simulink model "HEV_Model_Local_Solver"  (R2015a)
settings: Solver=ode23t  StartTime=0.0  StopTime=195  RelTol=1e-5  AbsTol=1e-4
PreLoadFcn:
  | load UrbanCycle1
  | load UrbanCycle2
  | load UrbanCycle3
  | load UrbanCycle4
  | load UrbanCycle5
  | 
  | assignin('base','decimation',1)
  | Pbatt = 21e3;
  | Vbatt =100;
  | Ts = 6e-5;   % time step
  | 
  | Drive_Cycle_Num = 1;
PostLoadFcn:
  | warning off Simulink:SL_UsingDefaultMaxStepSize
  | warning off Simulink:blocks:MatchingGotoNotFound
  | warning off Simulink:blocks:MatchingFromNotFound
  | warning off Simulink:blocks:TDelayBufferTooSmall
  | warning off Simulink:SL_SaveWithParameterizedLinks_Warning
  | warning off Simulink:SL_TDelayBufferTooSmall
  | warning off ne_sli:nesl_compile:SolverNotRecommended
  | warning off Simulink:SL_OutputNotConnected
  | warning off Simulink:SL_SetParamLinkChangeWarn
  | warning off Simulink:Engine:SaveWithDisabledLinks_Warning
  | warning('off','Simulink:SL_UINotUpdatedDuringRapidAccelSim');
  | warning off Simulink:Engine:OutputNotConnected
  | warning off Simulink:Engine:UINotUpdatedDuringRapidAccelSim
  | warning off Simulink:Engine:SaveWithParameterizedLinks_Warning
  | warning off Simulink:Engine:SolverMaskedZC
  | set_param(bdroot,'MaskedZcDiagnostic','none');
  | warning off Simulink:Engine:SolverInconsistentInitialConditionsWarnForDAE
  | set_param(bdroot,'IgnoredZcDiagnostic','none');
  | warning off Simulink:Engine:SolverIgnoredZCBracketing
  | set_param(bdroot,'MaxConsecutiveZCsMsg','none');
  | warning off Simulink:Engine:SolverConsecutiveZCNum
  | warning off Simulink:Engine:SolverMinStepSizeWarnForDAE
  | warning off Simulink:blocks:TDelayFixedBuffer
  | warning off Simulink:Engine:ExtModeCantUploadDataConstantSampleTime
  | warning off Simulink:tools:extModeOpenXPCWarning
  | warning off xPCTarget:sampleTime:sampleTimeInvariance
  | 
  | 
  | %Setup_HEV_Model_Configurations
InitFcn:
  | %Configure_HEV_Simulation
StartFcn:
  | tic;
StopFcn:
  | Elapsed_Sim_Time = toc; disp(['Elapsed time is ' num2str(Elapsed_Sim_Time)]); disp(['Fuel Used: ' num2str(FuelUsedLiters) ' Liters']); disp(' ');
model workspace (MAT data in the model file):
  guiH = 18054.0001221
undefined symbols (not defined in the file or in its folder): drive_block, drive_enginemodel, HEV_Param, sigbuilder_block, speed, torque
libraries: fl_lib x73, nesl_utility x31, sdl_lib x2, elec_lib x2, simulink x1, HEV_Battery_Lib x1, HEV_Vehicle_Dynamics_Lib x1, powerlib x1, slrtlib x1
(part 2 of 2)

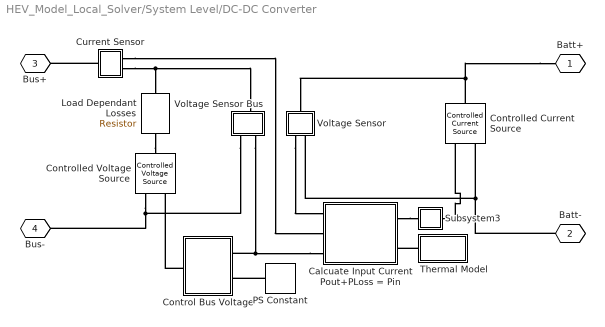
== system HEV_Model_Local_Solver/System Level/DC-DC Converter ==
  Calcuate Input Current Pout+PLoss = Pin : Subsystem
  Control Bus Voltage : Subsystem
  Controlled Current Source : fl_lib/Electrical/Electrical Sources/Controlled Current Source
  Controlled Voltage Source : fl_lib/Electrical/Electrical Sources/Controlled Voltage Source
  Current Sensor : Subsystem
  Load Dependant Losses : fl_lib/Electrical/Electrical Elements/Resistor  R=RLoadLoss Ohm  i_specify=off  i_priority=High  i=0 A  v_specify=off  v_priority=High  v=0 V
  PS Constant : fl_lib/Physical Signals/Sources/PS Constant  constant=Vout
  Subsystem3 : Subsystem
      mask Display: disp('S')
  Thermal Model : Subsystem
  Voltage Sensor : Subsystem
  Voltage Sensor Bus : Subsystem
  " Batt+" : PMIOPort  Tag=PMCPort  Port=1  Side=Left
  " Batt-" : PMIOPort  Tag=PMCPort  Port=2  Side=Left
  " Bus+" : PMIOPort  Tag=PMCPort  Port=3  Side=Right
  " Bus-" : PMIOPort  Tag=PMCPort  Port=4  Side=Right
  connections:
  Thermal Model/LConn1 -- Calcuate Input Current Pout+PLoss = Pin/RConn2
  Calcuate Input Current Pout+PLoss = Pin/LConn3 -- Control Bus Voltage/LConn1 -- Voltage Sensor Bus/RConn2
  Subsystem3/LConn1 -- Controlled Current Source/RConn1
  PS Constant/RConn1 -- Control Bus Voltage/LConn2
  Control Bus Voltage/RConn1 -- Controlled Voltage Source/RConn1
  " Batt+"/RConn1 -- Controlled Current Source/LConn1 -- Voltage Sensor/LConn1
  " Batt-"/RConn1 -- Controlled Current Source/RConn2 -- Voltage Sensor/RConn2
  Load Dependant Losses/RConn1 -- Controlled Voltage Source/LConn1
  " Bus-"/RConn1 -- Controlled Voltage Source/RConn2 -- Voltage Sensor Bus/RConn1
  Current Sensor/LConn1 -- " Bus+"/RConn1
  Current Sensor/RConn2 -- Load Dependant Losses/LConn1 -- Voltage Sensor Bus/LConn1
  Voltage Sensor/RConn1 -- Calcuate Input Current Pout+PLoss = Pin/LConn1
  Current Sensor/RConn1 -- Calcuate Input Current Pout+PLoss = Pin/LConn2
  Calcuate Input Current Pout+PLoss = Pin/RConn1 -- Subsystem3/RConn1

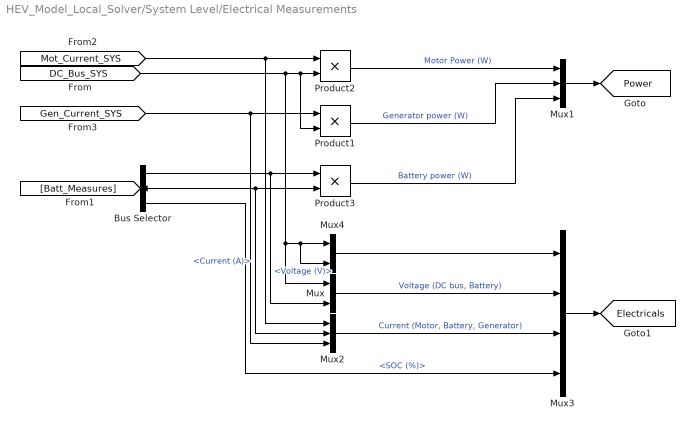
== system HEV_Model_Local_Solver/System Level/Electrical Measurements ==
  Bus Selector : BusSelector  OutputSignals=Voltage (V),Current (A),SOC (%)
  Mux : Mux  Inputs=2
  Mux1 : Mux  Inputs=3
  Mux2 : Mux  Inputs=3
  Mux3 : Mux
  Mux4 : Mux  Inputs=2
  Product1 : Product  RndMeth=Zero
  Product2 : Product  RndMeth=Zero
  Product3 : Product  RndMeth=Zero
  tag scope: Electricals=global, Power=global
  wires:
  Product2/1 -> Mux1/1  "Motor Power (W)"
  Product1/1 -> Mux1/2  "Generator power (W)"
  Product3/1 -> Mux1/3  "Battery power (W)"
  [Mot_Current_SYS] -> Product2/1, Mux2/1
  Mux1/1 -> [Power]
  [Batt_Measures] -> Bus Selector/1
  Bus Selector/1 -> Mux/2, Product3/1  "<Voltage (V)>"
  Bus Selector/2 -> Product3/2, Mux2/2  "<Current (A)>"
  Mux/1 -> Mux3/2  "Voltage (DC bus, Battery)"
  Mux2/1 -> Mux3/3  "Current (Motor, Battery, Generator)"
  [Gen_Current_SYS] -> Product1/1, Mux2/3
  Bus Selector/3 -> Mux3/4  "<SOC (%)>"
  [DC_Bus_SYS] -> Product2/2, Product1/2, Mux/1, Mux4/1, Mux4/2
  Mux3/1 -> [Electricals]
  Mux4/1 -> Mux3/1

== system HEV_Model_Local_Solver/System Level/Generator, Drive Measurements ==
  Constant1 : Constant  Value=0
  Constant2 : Constant  Value=0
  Mux1 : Mux
  Mux2 : Mux
  tag scope: GeneratorDrive=global, MotorDrive=global
  wires:
  [Mot_RPM_SYS] -> Mux2/2
  [Mot_TReq_SYS] -> Mux2/4, Mux2/3
  Mux2/1 -> [MotorDrive]
  Constant2/1 -> Mux2/1
  [Gen_RPM_SYS] -> Mux1/2
  [Gen_TReq_SYS] -> Mux1/3, Mux1/4
  Mux1/1 -> [GeneratorDrive]
  Constant1/1 -> Mux1/1

== system HEV_Model_Local_Solver/System Level/Speed Sensor1 ==
  Ideal Rotational Motion Sensor : fl_lib/Mechanical/Mechanical Sensors/Ideal Rotational Motion Sensor  offset=0 rad
  Mechanical Rotational Reference : fl_lib/Mechanical/Rotational Elements/Mechanical Rotational Reference
  PS-Simulink Converter : nesl_utility/PS-Simulink Converter  PhysicalDomain=network_engine_domain  SubClassName=ps_output  LeftPortType=input  RightPortType=output  PseudoPeriodic=off  Frequencies=[]  Unit=rpm  AffineConversion=off
  Sh : PMIOPort  Port=1  Side=Left
  Sh1 : PMIOPort  Port=2  Side=Right
  tag scope: Mot_RPM_SYS=global
  wires:
  PS-Simulink Converter/1 -> [Mot_RPM_SYS]  "Mot_RPM"
  connections:
  PS-Simulink Converter/LConn1 -- Ideal Rotational Motion Sensor/RConn2
  Sh/RConn1 -- Ideal Rotational Motion Sensor/LConn1 -- Sh1/RConn1
  Ideal Rotational Motion Sensor/RConn1 -- Mechanical Rotational Reference/LConn1

== system HEV_Model_Local_Solver/System Level/Speed Sensor2 ==
  Ideal Rotational Motion Sensor : fl_lib/Mechanical/Mechanical Sensors/Ideal Rotational Motion Sensor  offset=0 rad
  Mechanical Rotational Reference : fl_lib/Mechanical/Rotational Elements/Mechanical Rotational Reference
  PS-Simulink Converter : nesl_utility/PS-Simulink Converter  PhysicalDomain=network_engine_domain  SubClassName=ps_output  LeftPortType=input  RightPortType=output  PseudoPeriodic=off  Frequencies=[]  Unit=rpm  AffineConversion=off
  Sh : PMIOPort  Port=1  Side=Left
  Sh1 : PMIOPort  Port=2  Side=Right
  tag scope: Gen_RPM_SYS=global
  wires:
  PS-Simulink Converter/1 -> [Gen_RPM_SYS]  "Gen_RPM"
  connections:
  Ideal Rotational Motion Sensor/LConn1 -- Sh/RConn1 -- Sh1/RConn1
  PS-Simulink Converter/LConn1 -- Ideal Rotational Motion Sensor/RConn2
  Ideal Rotational Motion Sensor/RConn1 -- Mechanical Rotational Reference/LConn1

== system HEV_Model_Local_Solver/System Level/Synchronous Generator & Drive ==
  note: Note that the generator can turn backwards - this happens when accelerating from rest. The
      | generator also acts as a starter for the engine. If the engine is running, then the generator
      | controller is used to manage battery charging using torque-control mode, otherwise the
      | generator controller controls generator speed.
  TReq : Inport
  Calculate mechanical power & torque : Subsystem
      mask Display: disp('S')
  Calculate power : Subsystem
      mask Display: disp('S')
  GF : Subsystem
      mask Display: disp('GF')
  Inertia : fl_lib/Mechanical/Rotational Elements/Inertia  inertia=HEV_Param.Generator.Shaft_Inertia kg*m^2  w_specify=on  w_priority=High  w=0 rad/s  t_specify=off  t_priority=High  t=0 N*m
  Mechanical Rotational Reference : fl_lib/Mechanical/Rotational Elements/Mechanical Rotational Reference
  PS Terminator : Subsystem
      mask Display:
      | plot([0 0.9],[0.5 0.5]);
      | plot([0.5 0.9],[0.3 0.3]);
      | plot([0.5 0.9],[0.7 0.7]);
      | plot([0.9 0.9],[0.7 0.3]);
  Servomotor : elec_lib/Actuators & Drivers/Rotational Actuators/Servomotor  torque_speed_param=1  w_t=HEV_Param.Generator.TorqSpdLUT.SpeedRPM rpm  T_t=HEV_Param.Generator.TorqSpdLUT.TorqueNm N*m  torque_max=0.1 N*m  power_max=30 W  Tc=HEV_Param.Generator.TorqueControl_TimeConst s  eff=90  w_eff=2000 rpm  T_eff=200 N*m  Piron=0 W  Pbase=HEV_Param.Generator.TorqIndep_Elec_Loss W  Res=HEV_Param.Generator.Series_Resistance Ohm  J=0 kg*m^2  lam=HEV_Param.Generator.Damping N*m/(rad/s)  speed0=0 rpm  alpha=0.00393 1/K  Tmeas=25 C  thermal_mass=100 J/K  initial_temperature=25 C
  Vcc : PMIOPort  Port=1  Side=Right
  Gnd : PMIOPort  Port=2  Side=Right
  Shaft : PMIOPort  Port=3  Side=Right
  wires:
  TReq/1 -> GF/1(In1)
  connections:
  Shaft/RConn1 -- Inertia/LConn1 -- Calculate mechanical power & torque/RConn1
  Calculate power/LConn2 -- Servomotor/RConn1 -- Gnd/RConn1
  Vcc/RConn1 -- Calculate power/LConn1
  Calculate power/RConn1 -- Servomotor/LConn1
  GF/RConn1 -- Servomotor/LConn2
  PS Terminator/LConn1 -- Servomotor/RConn2
  Calculate mechanical power & torque/LConn1 -- Servomotor/LConn3
  Mechanical Rotational Reference/LConn1 -- Servomotor/RConn3

== system HEV_Model_Local_Solver/System Level/Synchronous Motor & Drive ==
  TReq : Inport
  Calculate electrical power : Subsystem
      mask Display: disp('S')
  Calculate mechanical power : Subsystem
      mask Display: disp('S')
  GF : Subsystem
      mask Display: disp('GF')
  Inertia : fl_lib/Mechanical/Rotational Elements/Inertia  inertia=HEV_Param.Motor.Shaft_Inertia kg*m^2  w_specify=on  w_priority=High  w=0 rad/s  t_specify=off  t_priority=High  t=0 N*m
  Mechanical Rotational Reference : fl_lib/Mechanical/Rotational Elements/Mechanical Rotational Reference
  PS Terminator1 : Subsystem
      mask Display:
      | plot([0 0.9],[0.5 0.5]);
      | plot([0.5 0.9],[0.3 0.3]);
      | plot([0.5 0.9],[0.7 0.7]);
      | plot([0.9 0.9],[0.7 0.3]);
  Servomotor : elec_lib/Actuators & Drivers/Rotational Actuators/Servomotor  torque_speed_param=1  w_t=HEV_Param.Motor.TorqSpdLUT.SpeedRPM rpm  T_t=HEV_Param.Motor.TorqSpdLUT.TorqueNm N*m  torque_max=0.1 N*m  power_max=30 W  Tc=HEV_Param.Motor.TorqueControl_TimeConst s  eff=HEV_Param.Motor.Efficiency  w_eff=2000 rpm  T_eff=200 N*m  Piron=0 W  Pbase=0 W  Res=HEV_Param.Motor.Series_Resistance Ohm  J=0 kg*m^2  lam=HEV_Param.Motor.Damping N*m/(rad/s)  speed0=0 rpm  alpha=0.00393 1/K  Tmeas=25 C  thermal_mass=100 J/K  initial_temperature=25 C
  Vcc : PMIOPort  Port=1  Side=Right
  Gnd : PMIOPort  Port=2  Side=Right
  Shaft : PMIOPort  Port=3  Side=Right
  wires:
  TReq/1 -> GF/1(In1)
  connections:
  Shaft/RConn1 -- Calculate mechanical power/RConn1 -- Inertia/LConn1
  PS Terminator1/LConn1 -- Servomotor/RConn2
  Calculate electrical power/LConn2 -- Gnd/RConn1 -- Servomotor/RConn1
  Vcc/RConn1 -- Calculate electrical power/LConn1
  Calculate electrical power/RConn1 -- Servomotor/LConn1
  GF/RConn1 -- Servomotor/LConn2
  Calculate mechanical power/LConn1 -- Servomotor/LConn3
  Servomotor/RConn3 -- Mechanical Rotational Reference/LConn1

== system HEV_Model_Local_Solver/System Level/Voltage sensor ==
  PS-Simulink Converter : nesl_utility/PS-Simulink Converter  PhysicalDomain=network_engine_domain  SubClassName=ps_output  LeftPortType=input  RightPortType=output  PseudoPeriodic=off  Frequencies=[]  Unit=V  AffineConversion=off
  Voltage Sensor : fl_lib/Electrical/Electrical Sensors/Voltage Sensor
  + : PMIOPort  Port=1  Side=Left
  - : PMIOPort  Port=2  Side=Right
  tag scope: DC_Bus_SYS=global
  wires:
  PS-Simulink Converter/1 -> [DC_Bus_SYS]
  connections:
  Voltage Sensor/RConn1 -- PS-Simulink Converter/LConn1
  +/RConn1 -- Voltage Sensor/LConn1
  -/RConn1 -- Voltage Sensor/RConn2

== system HEV_Model_Local_Solver/Control/Battery Charge Controller/Engine Model ==
  RPM : Inport
  Peak torque : Lookup  InputValues=speed  Table=torque  SaturateOnIntegerOverflow=on
  Max Torque : Outport
  wires:
  Peak torque/1 -> Max Torque/1
  RPM/1 -> Peak torque/1

== system HEV_Model_Local_Solver/Control/Engine Speed Controller/Engine Running ==
  RPM_Dem : Inport
  ICE_Enable : Inport  Port=2
  Alternate Logic : Subsystem
  Select Logic : ManualSwitch
  Engine Running : Outport
  tag scope: engine_running=global
  wires:
  RPM_Dem/1 -> Alternate Logic/1(RPM Dem)
  ICE_Enable/1 -> Select Logic/2
  Alternate Logic/1(ICE Enable) -> Select Logic/1
  Select Logic/1 -> Engine Running/1, [engine_running]

== system HEV_Model_Local_Solver/Control/Generator Controller/Enable Torque Demand ==
  Gen_Enable : Inport
  TrqDemCtrl : Inport  Port=2
  20Hz Lowpass Filter : TransferFcn  Denominator=[1/(2*pi*20) 1]
  Product : Product  RndMeth=Zero
  Select Logic : ManualSwitch  CurrentSetting=0
  G_Trq_Dem : Outport
  wires:
  Gen_Enable/1 -> 20Hz Lowpass Filter/1
  TrqDemCtrl/1 -> Product/2, Select Logic/2
  20Hz Lowpass Filter/1 -> Product/1
  Select Logic/1 -> G_Trq_Dem/1
  Product/1 -> Select Logic/1

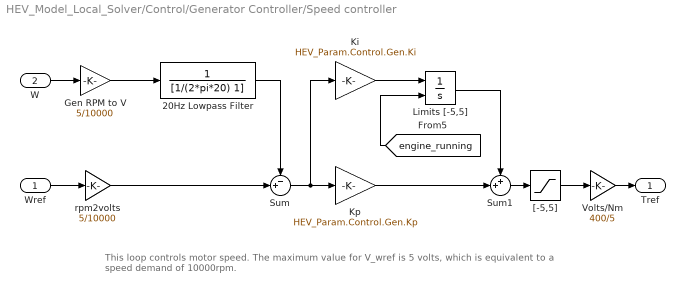
== system HEV_Model_Local_Solver/Control/Generator Controller/Speed controller ==
  note: This loop controls motor speed. The maximum value for V_wref is 5 volts,
      | which is equivalent to a speed demand of 10000rpm.
  Wref : Inport
  W : Inport  Port=2
  20Hz Lowpass Filter : TransferFcn  Denominator=[1/(2*pi*20) 1]
  Gen RPM to V : Gain  Gain=5/10000
  Ki : Gain  Gain=HEV_Param.Control.Gen.Ki
  Kp : Gain  Gain=HEV_Param.Control.Gen.Kp
  Limits [-5,5] : Integrator  ExternalReset=either  LimitOutput=on  UpperSaturationLimit=5  LowerSaturationLimit=-5
  Sum : Sum  Inputs=-+|
  Sum1 : Sum  Inputs=++|
  Volts/Nm : Gain  Gain=400/5
  "[-5,5]" : Saturate  UpperLimit=5  LowerLimit=-5
  rpm2volts : Gain  Gain=5/10000
  Tref : Outport
  wires:
  Sum/1 -> Ki/1, Kp/1
  [engine_running] -> Limits [-5,5]/2
  20Hz Lowpass Filter/1 -> Sum/1
  Limits [-5,5]/1 -> Sum1/1
  Kp/1 -> Sum1/2
  Ki/1 -> Limits [-5,5]/1
  Sum1/1 -> "[-5,5]"/1
  W/1 -> Gen RPM to V/1
  Wref/1 -> rpm2volts/1
  "[-5,5]"/1 -> Volts/Nm/1
  rpm2volts/1 -> Sum/2
  Gen RPM to V/1 -> 20Hz Lowpass Filter/1
  Volts/Nm/1 -> Tref/1

== system HEV_Model_Local_Solver/Control/Generator Controller/Subsystem1 ==
  In1 : Inport
  Gen_RPM_Dem : Outport
  tag scope: gen_rpm_dem=global
  wires:
  In1/1 -> Gen_RPM_Dem/1, [gen_rpm_dem]

== system HEV_Model_Local_Solver/Control/Motor Controller/Enable Torque Demand ==
  Mot_Enable : Inport
  TrqDemCtrl : Inport  Port=2
  20Hz Lowpass Filter : TransferFcn  Denominator=[1/(2*pi*10) 1]
  Product : Product  RndMeth=Zero
  Select Logic : ManualSwitch  CurrentSetting=0
  TrqDem : Outport
  wires:
  Mot_Enable/1 -> 20Hz Lowpass Filter/1
  TrqDemCtrl/1 -> Product/2, Select Logic/2
  Product/1 -> Select Logic/1
  20Hz Lowpass Filter/1 -> Product/1
  Select Logic/1 -> TrqDem/1

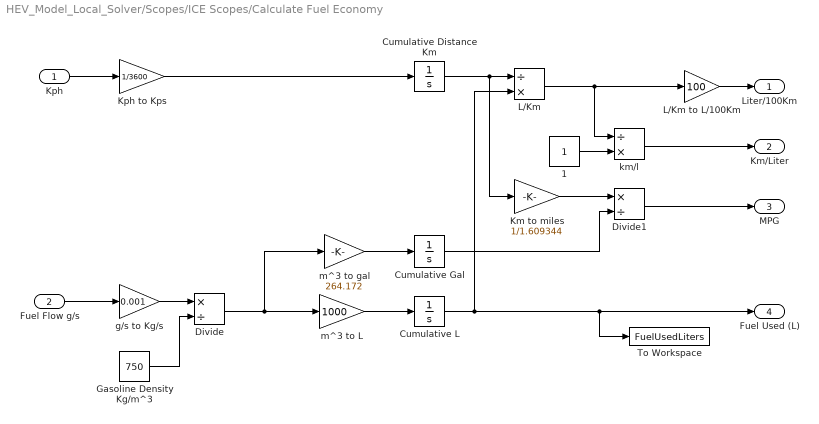
== system HEV_Model_Local_Solver/Scopes/ICE Scopes/Calculate Fuel Economy ==
  Kph : Inport
  Fuel Flow g/s : Inport  Port=2
  1 : Constant
  Cumulative Distance Km : Integrator  InitialCondition=eps
  Cumulative Gal : Integrator  InitialCondition=eps
  Cumulative L : Integrator  InitialCondition=eps
  Divide : Product  Inputs=*/
  Divide1 : Product  Inputs=*/
  Gasoline Density Kg/m^3 : Constant  Value=750
  Km to miles : Gain  Gain=1/1.609344
  Kph to Kps : Gain  Gain=1/3600
  L/Km : Product  Inputs=/*
  L/Km to L/100Km : Gain  Gain=100
  To Workspace : ToWorkspace  VariableName=FuelUsedLiters  SampleTime=-1
      settings: MaxDataPoints=1
  g/s to Kg/s : Gain  Gain=0.001
  km/l : Product  Inputs=/*
  m^3 to L : Gain  Gain=1000
  m^3 to gal : Gain  Gain=264.172
  Liter/100Km : Outport
  Km/Liter : Outport  Port=2
  MPG : Outport  Port=3
  Fuel Used (L) : Outport  Port=4
  wires:
  km/l/1 -> Km/Liter/1
  1/1 -> km/l/2
  Divide1/1 -> MPG/1
  L/Km to L/100Km/1 -> Liter/100Km/1
  Fuel Flow g/s/1 -> g/s to Kg/s/1
  Kph/1 -> Kph to Kps/1
  Cumulative Gal/1 -> Divide1/2
  Km to miles/1 -> Divide1/1
  L/Km/1 -> km/l/1, L/Km to L/100Km/1
  Cumulative Distance Km/1 -> Km to miles/1, L/Km/1
  Cumulative L/1 -> L/Km/2, Fuel Used (L)/1, To Workspace/1
  Kph to Kps/1 -> Cumulative Distance Km/1
  m^3 to gal/1 -> Cumulative Gal/1
  m^3 to L/1 -> Cumulative L/1
  Divide/1 -> m^3 to gal/1, m^3 to L/1
  Gasoline Density Kg/m^3/1 -> Divide/2
  g/s to Kg/s/1 -> Divide/1

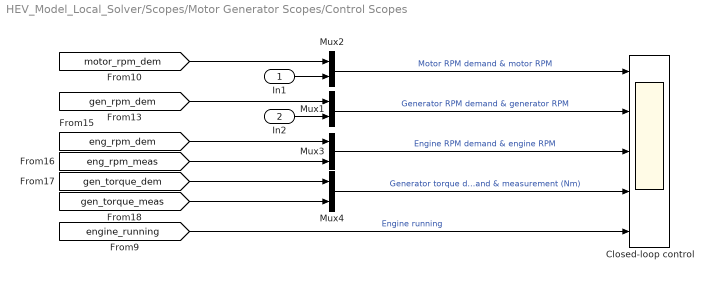
== system HEV_Model_Local_Solver/Scopes/Motor Generator Scopes/Control Scopes ==
  In1 : Inport
  In2 : Inport  Port=2
  Closed-loop control : Scope  NumInputPorts=5
      settings: TimeRange=30  YMin=0~-1000~0~-100~-0.1  YMax=600~3000~1500~100~1.1  SaveName=ScopeData5  MaxDataPoints=100  Decimation=decimation
  Mux{1..4} (4 alike) : Mux  Inputs=2
  wires:
  [motor_rpm_dem] -> Mux2/1
  Mux2/1 -> Closed-loop control/1  "Motor RPM demand & motor RPM"
  [gen_rpm_dem] -> Mux1/1
  Mux1/1 -> Closed-loop control/2  "Generator RPM demand & generator RPM"
  [eng_rpm_dem] -> Mux3/1
  [eng_rpm_meas] -> Mux3/2
  Mux3/1 -> Closed-loop control/3  "Engine RPM demand & engine RPM"
  [gen_torque_dem] -> Mux4/1
  [gen_torque_meas] -> Mux4/2
  Mux4/1 -> Closed-loop control/4  "Generator torque demand & measurement (Nm)"
  [engine_running] -> Closed-loop control/5  "Engine running"
  In1/1 -> Mux2/2
  In2/1 -> Mux1/2

== system HEV_Model_Local_Solver/System Level/DC-DC Converter/Calcuate Input Current Pout+PLoss = Pin ==
  note: Total Power
  note: Power Output
  Input^2 : fl_lib/Physical Signals/Functions/PS Math Function  fcn_choice=7
  No Div By 0 : fl_lib/Physical Signals/Nonlinear Operators/PS Max
  PS Add : fl_lib/Physical Signals/Functions/PS Add
  PS Constant : fl_lib/Physical Signals/Sources/PS Constant  constant=HEV_Param.DCDCConv.MinVin
  PS Divide : fl_lib/Physical Signals/Functions/PS Divide
  PS Product : fl_lib/Physical Signals/Functions/PS Product
  RLoadLoss : fl_lib/Physical Signals/Functions/PS Gain  gain=RLoadLoss
  V_In : PMIOPort  Port=1  Side=Left
  Iout : PMIOPort  Port=2  Side=Left
  Vout : PMIOPort  Port=3  Side=Left
  I_Input : PMIOPort  Port=4  Side=Right
  P Loss : PMIOPort  Port=5  Side=Right
  connections:
  PS Add/RConn1 -- PS Divide/LConn1
  No Div By 0/RConn1 -- PS Divide/LConn2
  V_In/RConn1 -- No Div By 0/LConn2
  No Div By 0/LConn1 -- PS Constant/RConn1
  P Loss/RConn1 -- RLoadLoss/RConn1 -- PS Add/LConn1
  PS Add/LConn2 -- PS Product/RConn1
  RLoadLoss/LConn1 -- Input^2/RConn1
  Iout/RConn1 -- PS Product/LConn1 -- Input^2/LConn1
  Vout/RConn1 -- PS Product/LConn2
  I_Input/RConn1 -- PS Divide/RConn1

== system HEV_Model_Local_Solver/System Level/DC-DC Converter/Control Bus Voltage ==
  Ki : fl_lib/Physical Signals/Functions/PS Gain  gain=Ki
  Kp : fl_lib/Physical Signals/Functions/PS Gain  gain=Kp
  PS Add1 : fl_lib/Physical Signals/Functions/PS Add
  PS Integrator : fl_lib/Physical Signals/Linear Operators/PS Integrator  x0=Vout
  PS Subtract : fl_lib/Physical Signals/Functions/PS Subtract
  Vmeas : PMIOPort  Port=1  Side=Left
  Vref : PMIOPort  Port=2  Side=Left
  VBus : PMIOPort  Port=3  Side=Right
  connections:
  PS Integrator/RConn1 -- PS Add1/LConn1
  PS Add1/LConn2 -- Kp/RConn1
  Kp/LConn1 -- PS Subtract/RConn1 -- Ki/LConn1
  PS Integrator/LConn1 -- Ki/RConn1
  Vmeas/RConn1 -- PS Subtract/LConn2
  Vref/RConn1 -- PS Subtract/LConn1
  VBus/RConn1 -- PS Add1/RConn1

== system HEV_Model_Local_Solver/System Level/DC-DC Converter/Current Sensor ==
  Current Sensor : fl_lib/Electrical/Electrical Sensors/Current Sensor
  PS-Simulink Converter : nesl_utility/PS-Simulink Converter  PhysicalDomain=network_engine_domain  SubClassName=ps_output  LeftPortType=input  RightPortType=output  PseudoPeriodic=off  Frequencies=[]  Unit=1  AffineConversion=off
  I : PMIOPort  Port=1  Side=Right
  + : PMIOPort  Port=2  Side=Left
  - : PMIOPort  Port=3  Side=Right
  tag scope: I_out=global
  wires:
  PS-Simulink Converter/1 -> [I_out]
  connections:
  -/RConn1 -- Current Sensor/RConn2
  +/RConn1 -- Current Sensor/LConn1
  PS-Simulink Converter/LConn1 -- I/RConn1 -- Current Sensor/RConn1

== system HEV_Model_Local_Solver/System Level/DC-DC Converter/Subsystem3 ==
  PS-Simulink Converter : nesl_utility/PS-Simulink Converter  PhysicalDomain=network_engine_domain  SubClassName=ps_output  LeftPortType=input  RightPortType=output  PseudoPeriodic=off  Frequencies=[]  Unit=1  AffineConversion=off
  Out : PMIOPort  Tag=PMCPort  Port=1  Side=Right
  In : PMIOPort  Tag=PMCPort  Port=2  Side=Left
  tag scope: I_in=global
  wires:
  PS-Simulink Converter/1 -> [I_in]
  connections:
  In/RConn1 -- Out/RConn1 -- PS-Simulink Converter/LConn1

== system HEV_Model_Local_Solver/System Level/DC-DC Converter/Thermal Model ==
  Air Temperature : fl_lib/Physical Signals/Sources/PS Constant  constant=HEV_Param.DCDCConv.Air_Temperature
  Ideal Heat Flow Source : fl_lib/Thermal/Thermal Sources/Ideal Heat Flow Source
  Ideal Temperature Source : fl_lib/Thermal/Thermal Sources/Ideal Temperature Source
  Nominal Case-Atmosphere Convective Heat Transfer : fl_lib/Thermal/Thermal Elements/Convective Heat Transfer  area=HEV_Param.DCDCConv.Convection.Area cm^2  heat_tr_coeff=HEV_Param.DCDCConv.Convection.HT_Coefficient W/(m^2 * K)  Q_specify=off  Q_priority=High  Q=0 J/s  T_specify=off  T_priority=High  T=0 K
  PtoHeat : fl_lib/Physical Signals/Functions/PS Gain  gain=HEV_Param.DCDCConv.EPower2Heat
  Subsystem : Subsystem
      mask Display: disp('S');
  Temperature Sensor : Subsystem
      mask Display:
      | patch([294.730220921338;294.546109275896;293.995547435362;293.083837611228;291.819760067491;290.215488561913;288.286473106077;286.051291173329;283.531468787557;280.75127321581;277.737479261253;274.519111407178;271.127164295357;267.594304230703;263.954554586898;260.242968142701;256.495289504528;252.747610866356;249.036024422158;245.396274778353;241.8634147137;238.471467601878;235.253099747803;232.239305793246;229.459110221499;226.939287835727;224.704105902979;222.775090447143;221.170818941565;219.906741397828;218.995031573694;218.44446973316;218.260358087718;218.44446973316;218.995031573694;219.906741397828;221.170818941565;222.775090447143;224.704105902979;226.939287835727;229.459110221499;232.239305793247;235.253099747803;238.471467601878;241.8634147137;245.396274778353;249.036024422158;252.747610866356;256.495289504528;260.242968142701;263.954554586898;267.594304230703;271.127164295357;274.519111407178;277.737479261253;280.75127321581;283.531468787557;286.051291173329;288.286473106077;290.215488561913;291.819760067491;293.083837611228;293.995547435362;294.546109275896;294.730220921338;294.730220921338], [122.389574535191;118.641895897019;114.930309452821;111.290559809016;107.757699744363;104.365752632541;101.147384778466;98.1335908239095;95.3533952521624;92.8335728663899;90.598390933642;88.6693754778057;87.0651039722279;85.8010264284914;84.8893166043572;84.3387547638233;84.1546431183815;84.3387547638233;84.8893166043572;85.8010264284914;87.0651039722279;88.6693754778058;90.598390933642;92.83357286639;95.3533952521625;98.1335908239095;101.147384778466;104.365752632541;107.757699744363;111.290559809016;114.930309452821;118.641895897019;122.389574535191;126.137253173364;129.848839617561;133.488589261366;137.02144932602;140.413396437841;143.631764291917;146.645558246473;149.42575381822;151.945576203992;154.18075813674;156.109773592576;157.714045098154;158.978122641891;159.889832466025;160.440394306559;160.624505952001;160.440394306559;159.889832466025;158.978122641891;157.714045098154;156.109773592576;154.18075813674;151.945576203992;149.42575381822;146.645558246473;143.631764291917;140.413396437841;137.02144932602;133.488589261366;129.848839617561;126.137253173364;122.389574535191;122.389574535191], [0;0;0])
      | plot([294.730220921338;294.546109275896;293.995547435362;293.083837611228;291.819760067491;290.215488561913;288.286473106077;286.051291173329;283.531468787557;280.75127321581;277.737479261253;274.519111407178;271.127164295357;267.594304230703;263.954554586898;260.242968142701;256.495289504528;252.747610866356;249.036024422158;245.396274778353;241.8634147137;238.471467601878;235.253099747803;232.239305793246;229.459110221499;226.939287835727;224.704105902979;222.775090447143;221.170818941565;219.906741397828;218.995031573694;218.44446973316;218.260358087718;218.44446973316;218.995031573694;219.906741397828;221.170818941565;222.775090447143;224.704105902979;226.939287835727;229.459110221499;232.239305793247;235.253099747803;238.471467601878;241.8634147137;245.396274778353;249.036024422158;252.747610866356;256.495289504528;260.242968142701;263.954554586898;267.594304230703;271.127164295357;274.519111407178;277.737479261253;280.75127321581;283.531468787557;286.051291173329;288.286473106077;290.215488561913;291.819760067491;293.083837611228;293.995547435362;294.546109275896;294.730220921338;294.730220921338], [122.389574535191;118.641895897019;114.930309452821;111.290559809016;107.757699744363;104.365752632541;101.147384778466;98.1335908239095;95.3533952521624;92.8335728663899;90.598390933642;88.6693754778057;87.0651039722279;85.8010264284914;84.8893166043572;84.3387547638233;84.1546431183815;84.3387547638233;84.8893166043572;85.8010264284914;87.0651039722279;88.6693754778058;90.598390933642;92.83357286639;95.3533952521625;98.1335908239095;101.147384778466;104.365752632541;107.757699744363;111.290559809016;114.930309452821;118.641895897019;122.389574535191;126.137253173364;129.848839617561;133.488589261366;137.02144932602;140.413396437841;143.631764291917;146.645558246473;149.42575381822;151.945576203992;154.18075813674;156.109773592576;157.714045098154;158.978122641891;159.889832466025;160.440394306559;160.624505952001;160.440394306559;159.889832466025;158.978122641891;157.714045098154;156.109773592576;154.18075813674;151.945576203992;149.42575381822;146.645558246473;143.631764291917;140.413396437841;137.02144932602;133.488589261366;129.848839617561;126.137253173364;122.389574535191;122.389574535191])
      | plot([243.771309033036;263.613159768283;263.613159768283;243.771309033036;243.771309033036], [438.410416245461;438.410416245461;112.4371541664;112.4371541664;438.410416245461])
      | plot([510.219018906355;0;0;510.219018906355;510.219018906355], [509.274168871343;509.274168871343;0;0;509.274168871343])
      | ;
      | %color('red');
      | %port_label('LConn', 1,'A')
      | %port_label('RConn', 1,'B')
  Thermal Mass : fl_lib/Thermal/Thermal Elements/Thermal Mass  mass=HEV_Param.DCDCConv.Thermal_Mass kg  sp_heat=HEV_Param.DCDCConv.Specific_Heat J/kg/K  Q_specify=off  Q_priority=High  Q=0 J/s  T_specify=on  T_priority=High  T=HEV_Param.DCDCConv.Initial_Temperature C
  Thermal Reference : fl_lib/Thermal/Thermal Elements/Thermal Reference
  Thermal Reference1 : fl_lib/Thermal/Thermal Elements/Thermal Reference
  P Loss : PMIOPort  Port=1  Side=Left
  connections:
  Thermal Reference1/LConn1 -- Ideal Heat Flow Source/RConn2
  PtoHeat/LConn1 -- Subsystem/RConn1
  Subsystem/LConn1 -- P Loss/RConn1
  Air Temperature/RConn1 -- Ideal Temperature Source/RConn1
  Ideal Temperature Source/RConn2 -- Thermal Reference/LConn1
  PtoHeat/RConn1 -- Ideal Heat Flow Source/RConn1
  Ideal Heat Flow Source/LConn1 -- Thermal Mass/LConn1 -- Nominal Case-Atmosphere Convective Heat Transfer/RConn1 -- Temperature Sensor/LConn1
  Nominal Case-Atmosphere Convective Heat Transfer/LConn1 -- Ideal Temperature Source/LConn1

== system HEV_Model_Local_Solver/System Level/DC-DC Converter/Voltage Sensor ==
  PS-Simulink Converter : nesl_utility/PS-Simulink Converter  PhysicalDomain=network_engine_domain  SubClassName=ps_output  LeftPortType=input  RightPortType=output  PseudoPeriodic=off  Frequencies=[]  Unit=1  AffineConversion=off
  Voltage Sensor In : fl_lib/Electrical/Electrical Sensors/Voltage Sensor
  + : PMIOPort  Port=1  Side=Left
  V : PMIOPort  Port=2  Side=Right
  - : PMIOPort  Port=3  Side=Right
  tag scope: V_in=global
  wires:
  PS-Simulink Converter/1 -> [V_in]
  connections:
  PS-Simulink Converter/LConn1 -- Voltage Sensor In/RConn1 -- V/RConn1
  -/RConn1 -- Voltage Sensor In/RConn2
  +/RConn1 -- Voltage Sensor In/LConn1

== system HEV_Model_Local_Solver/System Level/DC-DC Converter/Voltage Sensor Bus ==
  PS-Simulink Converter : nesl_utility/PS-Simulink Converter  PhysicalDomain=network_engine_domain  SubClassName=ps_output  LeftPortType=input  RightPortType=output  PseudoPeriodic=off  Frequencies=[]  Unit=1  AffineConversion=off
  Voltage Sensor Out : fl_lib/Electrical/Electrical Sensors/Voltage Sensor
  + : PMIOPort  Port=1  Side=Left
  - : PMIOPort  Port=2  Side=Right
  V : PMIOPort  Port=3  Side=Right
  tag scope: V_out=global
  wires:
  PS-Simulink Converter/1 -> [V_out]
  connections:
  -/RConn1 -- Voltage Sensor Out/RConn2
  PS-Simulink Converter/LConn1 -- Voltage Sensor Out/RConn1 -- V/RConn1
  +/RConn1 -- Voltage Sensor Out/LConn1

== system HEV_Model_Local_Solver/System Level/Synchronous Generator & Drive/Calculate mechanical power & torque ==
  Ideal Rotational Motion Sensor : fl_lib/Mechanical/Mechanical Sensors/Ideal Rotational Motion Sensor  offset=0 rad
  Mechanical Rotational Reference1 : fl_lib/Mechanical/Rotational Elements/Mechanical Rotational Reference
  PS Product : fl_lib/Physical Signals/Functions/PS Product
  PS-Simulink Converter : nesl_utility/PS-Simulink Converter  PhysicalDomain=network_engine_domain  SubClassName=ps_output  LeftPortType=input  RightPortType=output  PseudoPeriodic=off  Frequencies=[]  Unit=1  AffineConversion=off
  PS-Simulink Converter3 : nesl_utility/PS-Simulink Converter  PhysicalDomain=network_engine_domain  SubClassName=ps_output  LeftPortType=input  RightPortType=output  PseudoPeriodic=off  Frequencies=[]  Unit=N*m  AffineConversion=off
  Torque Sensor : fl_lib/Mechanical/Mechanical Sensors/Ideal Torque Sensor
  W to kW : Gain  Gain=1/1000
  C : PMIOPort  Port=1  Side=Right
  R : PMIOPort  Port=2  Side=Left
  tag scope: Pm_genr=global, gen_torque_meas=global
  wires:
  PS-Simulink Converter/1 -> [gen_torque_meas]
  PS-Simulink Converter3/1 -> W to kW/1
  W to kW/1 -> [Pm_genr]
  connections:
  C/RConn1 -- Torque Sensor/RConn1
  R/RConn1 -- Torque Sensor/LConn1 -- Ideal Rotational Motion Sensor/LConn1
  PS Product/RConn1 -- PS-Simulink Converter3/LConn1
  PS-Simulink Converter/LConn1 -- PS Product/LConn1 -- Torque Sensor/RConn2
  Ideal Rotational Motion Sensor/RConn2 -- PS Product/LConn2
  Mechanical Rotational Reference1/LConn1 -- Ideal Rotational Motion Sensor/RConn1

== system HEV_Model_Local_Solver/System Level/Synchronous Generator & Drive/Calculate power ==
  Current Sensor : fl_lib/Electrical/Electrical Sensors/Current Sensor
  PS Product1 : fl_lib/Physical Signals/Functions/PS Product
  PS-Simulink Converter4 : nesl_utility/PS-Simulink Converter  PhysicalDomain=network_engine_domain  SubClassName=ps_output  LeftPortType=input  RightPortType=output  PseudoPeriodic=off  Frequencies=[]  Unit=N*m  AffineConversion=off
  Voltage Sensor : fl_lib/Electrical/Electrical Sensors/Voltage Sensor
  W to kW : Gain  Gain=1/1000
  + : PMIOPort  Port=1  Side=Left
  ref : PMIOPort  Port=2  Side=Left
  - : PMIOPort  Port=3  Side=Right
  tag scope: Pe_genr=global
  wires:
  W to kW/1 -> [Pe_genr]
  PS-Simulink Converter4/1 -> W to kW/1
  connections:
  Current Sensor/RConn1 -- PS Product1/LConn1
  -/RConn1 -- Current Sensor/RConn2 -- Voltage Sensor/LConn1
  Voltage Sensor/RConn1 -- PS Product1/LConn2
  PS-Simulink Converter4/LConn1 -- PS Product1/RConn1
  +/RConn1 -- Current Sensor/LConn1
  ref/RConn1 -- Voltage Sensor/RConn2

== system HEV_Model_Local_Solver/System Level/Synchronous Generator & Drive/GF ==
  In1 : Inport
  Simulink-PS Converter : nesl_utility/Simulink-PS Converter  PhysicalDomain=network_engine_domain  SubClassName=ps_input  LeftPortType=input  RightPortType=output  PseudoPeriodic=off  Frequencies=[]  NoiseDistribution=none  NoiseParameters=[]  Unit=1  AffineConversion=off  InputFiltering=off  SimscapeFilterOrder=1  InputFilterTimeConstant=.001  UdotUserProvided=0
  Shaft : PMIOPort  Port=1  Side=Right
  tag scope: Gen_TReq_SYS=global
  wires:
  In1/1 -> Simulink-PS Converter/1, [Gen_TReq_SYS]
  connections:
  Shaft/RConn1 -- Simulink-PS Converter/RConn1

== system HEV_Model_Local_Solver/System Level/Synchronous Generator & Drive/PS Terminator ==
  PS-Simulink Converter 2 : nesl_utility/PS-Simulink Converter  PhysicalDomain=network_engine_domain  SubClassName=ps_output  LeftPortType=input  RightPortType=output  PseudoPeriodic=off  Frequencies=[]  Unit=rpm  AffineConversion=off
  Terminator : Terminator
  R : PMIOPort  Port=1  Side=Left
  wires:
  PS-Simulink Converter 2/1 -> Terminator/1
  connections:
  R/RConn1 -- PS-Simulink Converter 2/LConn1

== system HEV_Model_Local_Solver/System Level/Synchronous Motor & Drive/Calculate electrical power ==
  Current Sensor : fl_lib/Electrical/Electrical Sensors/Current Sensor
  PS Product1 : fl_lib/Physical Signals/Functions/PS Product
  PS-Simulink Converter4 : nesl_utility/PS-Simulink Converter  PhysicalDomain=network_engine_domain  SubClassName=ps_output  LeftPortType=input  RightPortType=output  PseudoPeriodic=off  Frequencies=[]  Unit=N*m  AffineConversion=off
  Voltage Sensor : fl_lib/Electrical/Electrical Sensors/Voltage Sensor
  W to kW : Gain  Gain=1/1000
  + : PMIOPort  Port=1  Side=Left
  ref : PMIOPort  Port=2  Side=Left
  - : PMIOPort  Port=3  Side=Right
  tag scope: Pe_motor=global
  wires:
  PS-Simulink Converter4/1 -> W to kW/1
  W to kW/1 -> [Pe_motor]
  connections:
  ref/RConn1 -- Voltage Sensor/RConn2
  +/RConn1 -- Current Sensor/LConn1
  PS-Simulink Converter4/LConn1 -- PS Product1/RConn1
  Voltage Sensor/RConn1 -- PS Product1/LConn2
  Voltage Sensor/LConn1 -- Current Sensor/RConn2 -- -/RConn1
  Current Sensor/RConn1 -- PS Product1/LConn1

== system HEV_Model_Local_Solver/System Level/Synchronous Motor & Drive/Calculate mechanical power ==
  Ideal Rotational Motion Sensor : fl_lib/Mechanical/Mechanical Sensors/Ideal Rotational Motion Sensor  offset=0 rad
  Mechanical Rotational Reference1 : fl_lib/Mechanical/Rotational Elements/Mechanical Rotational Reference
  PS Product : fl_lib/Physical Signals/Functions/PS Product
  PS-Simulink Converter3 : nesl_utility/PS-Simulink Converter  PhysicalDomain=network_engine_domain  SubClassName=ps_output  LeftPortType=input  RightPortType=output  PseudoPeriodic=off  Frequencies=[]  Unit=N*m  AffineConversion=off
  Torque Sensor : fl_lib/Mechanical/Mechanical Sensors/Ideal Torque Sensor
  W to kW : Gain  Gain=1/1000
  C : PMIOPort  Port=1  Side=Right
  R : PMIOPort  Port=2  Side=Left
  tag scope: Pm_motor=global
  wires:
  W to kW/1 -> [Pm_motor]
  PS-Simulink Converter3/1 -> W to kW/1
  connections:
  Mechanical Rotational Reference1/LConn1 -- Ideal Rotational Motion Sensor/RConn1
  Ideal Rotational Motion Sensor/RConn2 -- PS Product/LConn2
  Torque Sensor/RConn2 -- PS Product/LConn1
  PS Product/RConn1 -- PS-Simulink Converter3/LConn1
  Ideal Rotational Motion Sensor/LConn1 -- Torque Sensor/LConn1 -- R/RConn1
  C/RConn1 -- Torque Sensor/RConn1

== system HEV_Model_Local_Solver/System Level/Synchronous Motor & Drive/GF ==
  In1 : Inport
  Simulink-PS Converter : nesl_utility/Simulink-PS Converter  PhysicalDomain=network_engine_domain  SubClassName=ps_input  LeftPortType=input  RightPortType=output  PseudoPeriodic=off  Frequencies=[]  NoiseDistribution=none  NoiseParameters=[]  Unit=1  AffineConversion=off  InputFiltering=off  SimscapeFilterOrder=1  InputFilterTimeConstant=.001  UdotUserProvided=0
  Conn1 : PMIOPort  Port=1  Side=Right
  tag scope: Mot_TReq_SYS=global
  wires:
  In1/1 -> Simulink-PS Converter/1, [Mot_TReq_SYS]
  connections:
  Simulink-PS Converter/RConn1 -- Conn1/RConn1

== system HEV_Model_Local_Solver/System Level/Synchronous Motor & Drive/PS Terminator1 ==
  PS-Simulink Converter 2 : nesl_utility/PS-Simulink Converter  PhysicalDomain=network_engine_domain  SubClassName=ps_output  LeftPortType=input  RightPortType=output  PseudoPeriodic=off  Frequencies=[]  Unit=rpm  AffineConversion=off
  Terminator : Terminator
  R : PMIOPort  Port=1  Side=Left
  wires:
  PS-Simulink Converter 2/1 -> Terminator/1
  connections:
  R/RConn1 -- PS-Simulink Converter 2/LConn1

== system HEV_Model_Local_Solver/Control/Engine Speed Controller/Engine Running/Alternate Logic ==
  RPM Dem : Inport
  Allow time for engine to start : TransportDelay
  No delay for engine stopping : Product  RndMeth=Zero
  Start engine : Fcn  Expr=u(1) > HEV_Param.Control.Engine_Start_RPM
  ICE Enable : Outport
  wires:
  Start engine/1 -> Allow time for engine to start/1, No delay for engine stopping/2
  Allow time for engine to start/1 -> No delay for engine stopping/1
  RPM Dem/1 -> Start engine/1
  No delay for engine stopping/1 -> ICE Enable/1

== system HEV_Model_Local_Solver/System Level/DC-DC Converter/Thermal Model/Subsystem ==
  PS-Simulink Converter1 : nesl_utility/PS-Simulink Converter  PhysicalDomain=network_engine_domain  SubClassName=ps_output  LeftPortType=input  RightPortType=output  PseudoPeriodic=off  Frequencies=[]  Unit=C  AffineConversion=on
  In : PMIOPort  Port=1  Side=Left
  Out : PMIOPort  Port=2  Side=Right
  tag scope: DCDC_Power_Loss=global
  wires:
  PS-Simulink Converter1/1 -> [DCDC_Power_Loss]
  connections:
  Out/RConn1 -- PS-Simulink Converter1/LConn1 -- In/RConn1

== system HEV_Model_Local_Solver/System Level/DC-DC Converter/Thermal Model/Temperature Sensor ==
  Ideal Temperature Sensor : fl_lib/Thermal/Thermal Sensors/Ideal Temperature Sensor
  PS-Simulink Converter : nesl_utility/PS-Simulink Converter  PhysicalDomain=network_engine_domain  SubClassName=ps_output  LeftPortType=input  RightPortType=output  PseudoPeriodic=off  Frequencies=[]  Unit=C  AffineConversion=on
  Thermal Reference : fl_lib/Thermal/Thermal Elements/Thermal Reference
  Conn2 : PMIOPort  Port=1  Side=Left
  tag scope: DCDC_SYS=global
  wires:
  PS-Simulink Converter/1 -> [DCDC_SYS]  "DCDC_Temp"
  connections:
  Conn2/RConn1 -- Ideal Temperature Sensor/LConn1
  Thermal Reference/LConn1 -- Ideal Temperature Sensor/RConn1
  PS-Simulink Converter/LConn1 -- Ideal Temperature Sensor/RConn2

== stateflow chart HEV_Model_Local_Solver/Control/Mode Logic ==
  settings: updateMethod=DISCRETE  sampleTime=HEV_Param.Control.Mode_Logic_TS
  state Motion_mode
    state Start_mode
      entry: Gen_Enable=1;
      Mot_Enable=1;
      ICE_Enable=0;
    state Normal_mode
      entry: ICE_Enable=1;
      state Accelerate_mode
        entry: Gen_Enable=0;
        Mot_Enable=1;
      state Cruise_mode
        entry: Mot_Enable=1;
        state charge
          entry:Gen_Enable=1;
        state nocharge
          entry:Gen_Enable=0;
        (default) -> charge
        charge -> nocharge : [charge>99.9]
        nocharge -> charge : [charge<30]
      (default) -> Accelerate_mode
      Cruise_mode -> Accelerate_mode : [(speed <0.998*oldspeed() ...
          | || speed>1.002*oldspeed()) ...
          | && charge>30]
      Accelerate_mode -> Cruise_mode : [(speed >0.998*oldspeed() ...
          |  && speed<1.002* ...
          | oldspeed())|| charge<=30]
    (default) -> Start_mode
    Normal_mode -> Start_mode : [engine_speed<=EngOffRPM]
    Start_mode -> Normal_mode : [engine_speed>EngOnRPM]
  state Brake_mode
    entry: Mot_Enable=1;
    Gen_Enable=0;
    ICE_Enable=0;
  (default) -> Motion_mode
  Motion_mode -> Brake_mode : [brake>=0.05]
  Brake_mode -> Motion_mode : [brake<0.05]
  data: y function_output double; speed input; Mot_Enable output double; Gen_Enable output double; brake input; speed_buffer local double size=21; ICE_Enable output double; charge input; engine_speed input; EngOnRPM constant double =HEV_Param.Control.Engine_Start_RPM; EngOffRPM constant double =HEV_Param.Control.Engine_Stop_RPM
  function y = oldspeed:
    | function y = oldspeed
    | speed_buffer(2:end) = speed_buffer(1:end-1);
    | speed_buffer(1) = speed;
    | y = mean(speed_buffer);
